simulink model "closedloop_3d"  (R2016b)
settings: Solver=FixedStepAuto  StartTime=0.0  StopTime=40  FixedStep=0.001  RelTol=1e-3
values from neighbouring files (symbols this model uses):
  C_psi = 3.1176e-5    (= 3.1176e-05)    [NL_1D_Model.m]    (also in NL_3D_Model.m)
  dead_time = 0.001    [NL_3D_Model.m]
  filter_select = 1    [NL_3D_Model.m]
  I_K_inv = inv(I_K)    [NL_3D_Model.m]
  I_R_inv = inv(I_R)    [NL_3D_Model.m]
  K = [ 0.0361, 1.0652, -1.1013, -0.6746, 0.3836, 0.1820, -0.0015, -0.0001, -0.0001 ... (first row only)    [NL_3D_Model.m]
  l_C = (l_M*m_r+l_AC*m_k)/m_g    [NL_1D_Model.m]    (also in NL_3D_Model.m = 0.066)
  m = m_r + m_k    (= 0.311)    [NL_1D_Model.m]    (also in NL_3D_Model.m = 1.532)
  T_comp = 2    [NL_3D_Model.m]
  Ta = 0.02    [NL_3D_Model.m]
  u_sat_on = true    [NL_3D_Model_u_limited.m]    (also in NL_3D_Model_u_limited_x_offset.m)
  x_0 = degtorad([3;0;0])    [NL_1D_Model.m]    (also in NL_3D_Model_u_limited.m = [x_0;zeros(6,1)]; NL_3D_Model_u_limited_x_offset.m = [x_0;zeros(6,1)])
  x_offset = zeros(9,1)    [NL_3D_Model_u_limited.m]    (also in NL_3D_Model_u_limited_x_offset.m = [0.05; 0.2; 0.5; zeros(6,1)])
libraries: vrlib x3, simulink x1
settings Model: Creator=michael  LastModifiedBy=michael

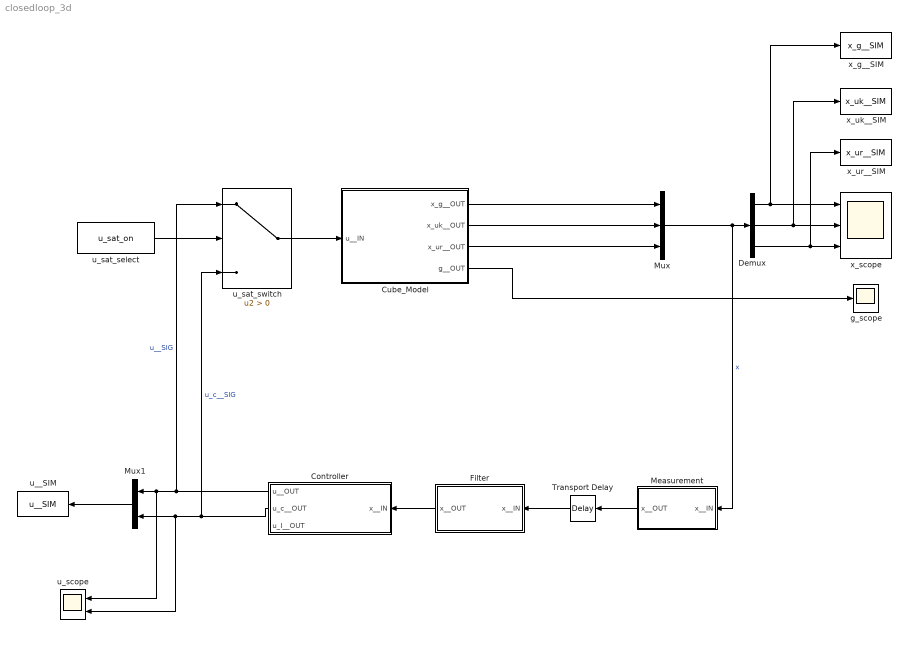
== system closedloop_3d ==
  Controller : Subsystem
  Cube_Model : Subsystem
  Demux : Demux  Outputs=3
  Filter : Subsystem
  Measurement : Subsystem
  Mux : Mux  Inputs=3
  Mux1 : Mux  Inputs=2
  Transport Delay : TransportDelay  DelayTime=dead_time  InitialOutput=x_0
  g_scope : Scope
  u__SIM : ToWorkspace  VariableName=u__SIM  SaveFormat=Timeseries  SampleTime=-1
  u_sat_select : Constant  Value=u_sat_on
  u_sat_switch : Switch  Criteria=u2 > Threshold
  u_scope : Scope  NumInputPorts=2
  x_g__SIM : ToWorkspace  VariableName=x_g__SIM  SaveFormat=Timeseries  SampleTime=-1
  x_scope : Scope  NumInputPorts=3
  x_uk__SIM : ToWorkspace  VariableName=x_uk__SIM  SaveFormat=Timeseries  SampleTime=-1
  x_ur__SIM : ToWorkspace  VariableName=x_ur__SIM  SaveFormat=Timeseries  SampleTime=-1
  wires:
  Cube_Model/1(x_g__OUT) -> Mux/1
  Cube_Model/2(x_uk__OUT) -> Mux/2
  Cube_Model/3(x_ur__OUT) -> Mux/3
  Mux/1 -> Measurement/1(x__IN), Demux/1  "x"
  Demux/3 -> x_ur__SIM/1, x_scope/3
  Demux/1 -> x_g__SIM/1, x_scope/1
  Demux/2 -> x_uk__SIM/1, x_scope/2
  Cube_Model/4(g__OUT) -> g_scope/1
  u_sat_select/1 -> u_sat_switch/2
  Mux1/1 -> u__SIM/1
  Controller/1(u__OUT) -> u_sat_switch/1, u_scope/1, Mux1/1  "u__SIG"
  Controller/2(u_c__OUT) -> u_sat_switch/3, u_scope/2, Mux1/2  "u_c__SIG"
  Filter/1(x__OUT) -> Controller/1(x__IN)
  Measurement/1(x__OUT) -> Transport Delay/1
  Transport Delay/1 -> Filter/1(x__IN)
  u_sat_switch/1 -> Cube_Model/1(u__IN)

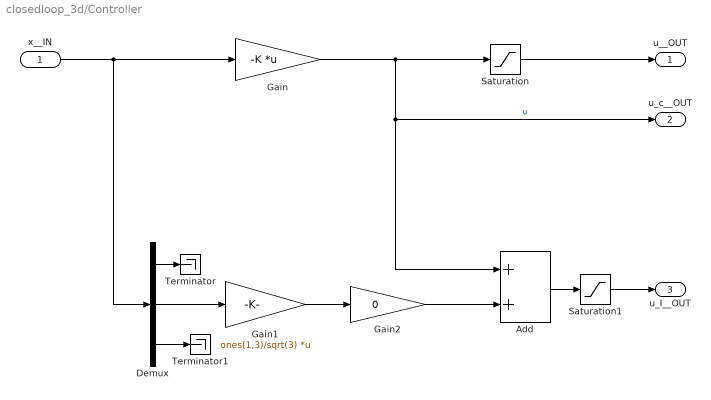
== system closedloop_3d/Controller ==
  x__IN : Inport  SampleTime=Ta
  Add : Sum
  Demux : Demux  Outputs=3
  Gain : Gain  Gain=-K  Multiplication=Matrix(K*u) (u vector)
  Gain1 : Gain  Gain=ones(1,3)/sqrt(3)  Multiplication=Matrix(K*u) (u vector)
  Gain2 : Gain  Gain=0
  Saturation : Saturate  UpperLimit=0.11  LowerLimit=-0.11
  Saturation1 : Saturate  UpperLimit=0.11  LowerLimit=-0.11
  Terminator : Terminator
  Terminator1 : Terminator
  u__OUT : Outport
  u_c__OUT : Outport  Port=2
  u_I__OUT : Outport  Port=3
  wires:
  x__IN/1 -> Demux/1, Gain/1
  Gain/1 -> Add/1, u_c__OUT/1, Saturation/1  "u"
  Saturation/1 -> u__OUT/1
  Demux/2 -> Gain1/1
  Demux/1 -> Terminator/1
  Gain1/1 -> Gain2/1
  Add/1 -> Saturation1/1
  Gain2/1 -> Add/2
  Saturation1/1 -> u_I__OUT/1
  Demux/3 -> Terminator1/1

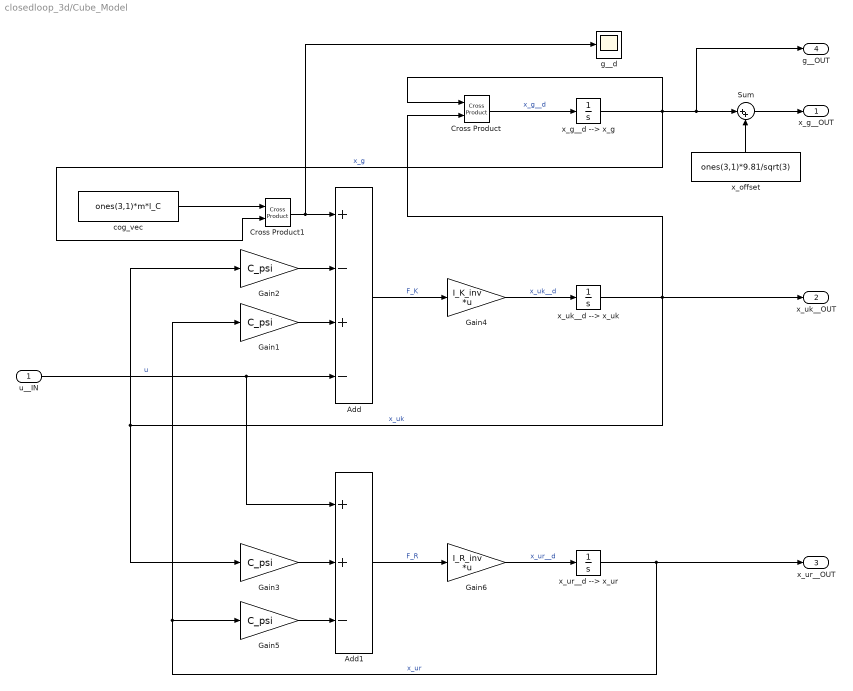
== system closedloop_3d/Cube_Model ==
  u__IN : Inport
  Add : Sum  Inputs=+-+-
  Add1 : Sum  Inputs=++-
  Cross Product : vrlib/Utilities/Cross Product
  Cross Product1 : vrlib/Utilities/Cross Product
  Gain{1..3,5} (4 alike) : Gain  Gain=C_psi
  Gain4 : Gain  Gain=I_K_inv  Multiplication=Matrix(K*u) (u vector)
  Gain6 : Gain  Gain=I_R_inv  Multiplication=Matrix(K*u) (u vector)
  Sum : Sum  Inputs=|++
  cog_vec : Constant  Value=ones(3,1)*m*l_C
  g__d : Scope
  x_g__d --> x_g : Integrator  InitialCondition=x_0(1:3)
  x_offset : Constant  Value=ones(3,1)*9.81/sqrt(3)
  x_uk__d --> x_uk : Integrator  InitialCondition=x_0(4:6)
  x_ur__d --> x_ur : Integrator  InitialCondition=x_0(7:9)
  x_g__OUT : Outport
  x_uk__OUT : Outport  Port=2
  x_ur__OUT : Outport  Port=3
  g__OUT : Outport  Port=4
  wires:
  Add/1 -> Gain4/1  "F_K"
  Gain5/1 -> Add1/3
  Gain4/1 -> x_uk__d --> x_uk/1  "x_uk__d"
  Gain1/1 -> Add/3
  Gain2/1 -> Add/2
  u__IN/1 -> Add1/1, Add/4  "u"
  Gain3/1 -> Add1/2
  x_ur__d --> x_ur/1 -> x_ur__OUT/1, Gain1/1, Gain5/1  "x_ur"
  Gain6/1 -> x_ur__d --> x_ur/1  "x_ur__d"
  Add1/1 -> Gain6/1  "F_R"
  x_g__d --> x_g/1 -> Cross Product1/2, g__OUT/1, Sum/1, Cross Product/1  "x_g"
  x_uk__d --> x_uk/1 -> x_uk__OUT/1, Cross Product/2, Gain3/1, Gain2/1  "x_uk"
  Cross Product/1 -> x_g__d --> x_g/1  "x_g__d"
  Sum/1 -> x_g__OUT/1
  x_offset/1 -> Sum/2
  cog_vec/1 -> Cross Product1/1
  Cross Product1/1 -> g__d/1, Add/1

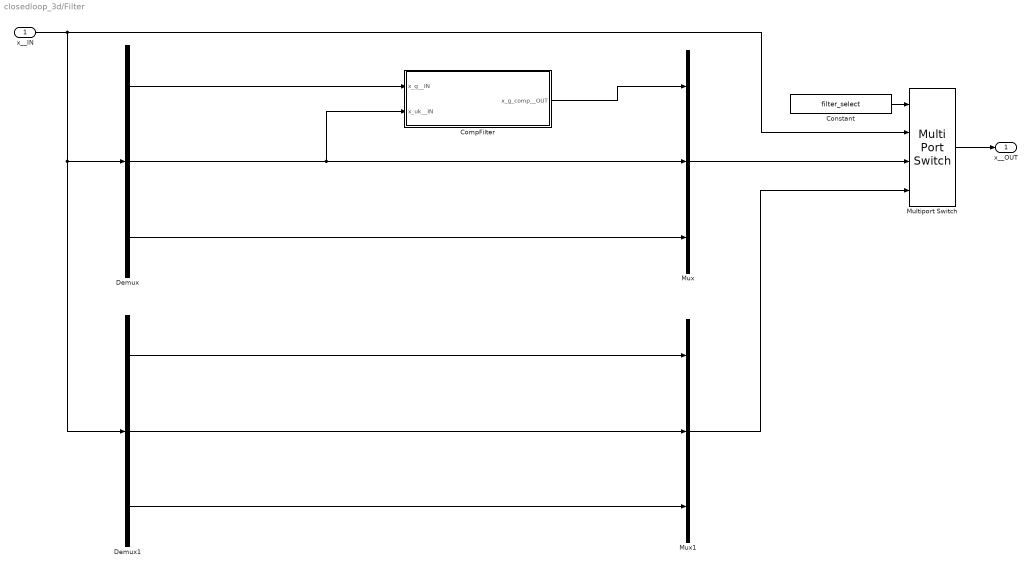
== system closedloop_3d/Filter ==
  x__IN : Inport  SampleTime=0.02
  CompFilter : Subsystem
  Constant : Constant  Value=filter_select
  Demux : Demux  Outputs=3
  Demux1 : Demux  Outputs=3
  Multiport Switch : MultiPortSwitch  DataPortOrder=Zero-based contiguous
  Mux : Mux  Inputs=3
  Mux1 : Mux  Inputs=3
  x__OUT : Outport
  wires:
  x__IN/1 -> Multiport Switch/2, Demux1/1, Demux/1
  Demux/2 -> Mux/2, CompFilter/2(x_uk__IN)
  Mux/1 -> Multiport Switch/3
  Demux/3 -> Mux/3
  CompFilter/1(x_g_comp__OUT) -> Mux/1
  Demux/1 -> CompFilter/1(x_g__IN)
  Demux1/1 -> Mux1/1
  Demux1/2 -> Mux1/2
  Demux1/3 -> Mux1/3
  Constant/1 -> Multiport Switch/1
  Multiport Switch/1 -> x__OUT/1
  Mux1/1 -> Multiport Switch/4

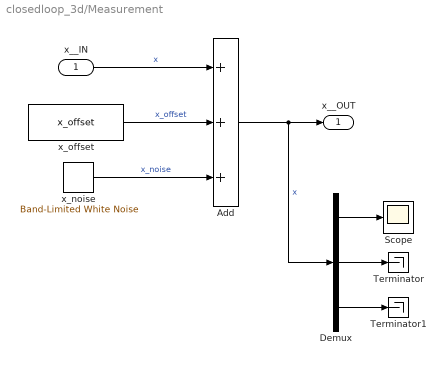
== system closedloop_3d/Measurement ==
  x__IN : Inport
  Add : Sum  Inputs=+++
  Demux : Demux  Outputs=3
  Scope : Scope
  Terminator : Terminator
  Terminator1 : Terminator
  x_noise : simulink/Sources/Band-Limited White Noise  Cov=x_noise  Ts=Ta  seed=[23341, 12324, 12341, 0, 0, 0, 0, 0, 0]
  x_offset : Constant  Value=x_offset
  x__OUT : Outport
  wires:
  x__IN/1 -> Add/1  "x"
  Add/1 -> Demux/1, x__OUT/1  "x"
  x_offset/1 -> Add/2  "x_offset"
  x_noise/1 -> Add/3  "x_noise"
  Demux/1 -> Scope/1
  Demux/2 -> Terminator/1
  Demux/3 -> Terminator1/1

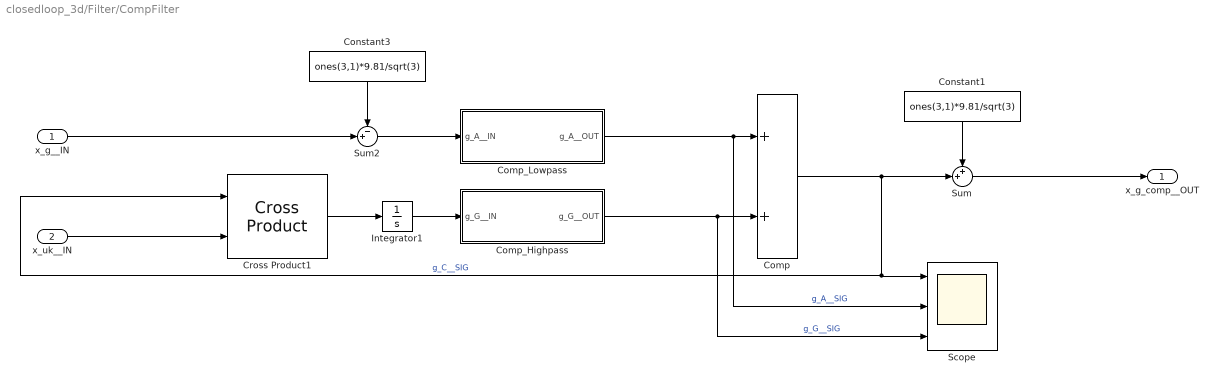
== system closedloop_3d/Filter/CompFilter ==
  x_g__IN : Inport
  x_uk__IN : Inport  Port=2
  Comp : Sum
  Comp_Highpass : Subsystem
  Comp_Lowpass : Subsystem
  Constant1 : Constant  Value=ones(3,1)*9.81/sqrt(3)
  Constant3 : Constant  Value=ones(3,1)*9.81/sqrt(3)
  Cross Product1 : vrlib/Utilities/Cross Product
  Integrator1 : Integrator  InitialCondition=x_0(1:3)
  Scope : Scope  NumInputPorts=3
  Sum : Sum  Inputs=++|
  Sum2 : Sum  Inputs=-+|
  x_g_comp__OUT : Outport
  wires:
  x_uk__IN/1 -> Cross Product1/2
  Comp_Lowpass/1(g_A__OUT) -> Scope/2, Comp/1  "g_A__SIG"
  Cross Product1/1 -> Integrator1/1
  Comp/1 -> Sum/2, Cross Product1/1, Scope/1  "g_C__SIG"
  Comp_Highpass/1(g_G__OUT) -> Scope/3, Comp/2  "g_G__SIG"
  Integrator1/1 -> Comp_Highpass/1(g_G__IN)
  x_g__IN/1 -> Sum2/2
  Sum2/1 -> Comp_Lowpass/1(g_A__IN)
  Constant3/1 -> Sum2/1
  Sum/1 -> x_g_comp__OUT/1
  Constant1/1 -> Sum/1

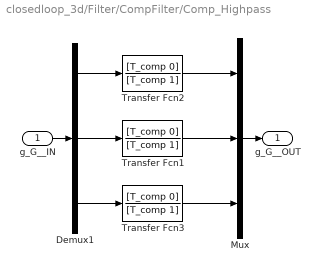
== system closedloop_3d/Filter/CompFilter/Comp_Highpass ==
  g_G__IN : Inport
  Demux1 : Demux  Outputs=3
  Mux : Mux  Inputs=3
  Transfer Fcn1 : TransferFcn  Numerator=[T_comp 0]  Denominator=[T_comp 1]
  Transfer Fcn2 : TransferFcn  Numerator=[T_comp 0]  Denominator=[T_comp 1]
  Transfer Fcn3 : TransferFcn  Numerator=[T_comp 0]  Denominator=[T_comp 1]
  g_G__OUT : Outport
  wires:
  Demux1/3 -> Transfer Fcn3/1
  g_G__IN/1 -> Demux1/1
  Transfer Fcn3/1 -> Mux/3
  Demux1/2 -> Transfer Fcn1/1
  Transfer Fcn1/1 -> Mux/2
  Mux/1 -> g_G__OUT/1
  Demux1/1 -> Transfer Fcn2/1
  Transfer Fcn2/1 -> Mux/1

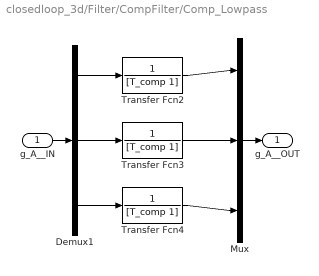
== system closedloop_3d/Filter/CompFilter/Comp_Lowpass ==
  g_A__IN : Inport
  Demux1 : Demux  Outputs=3
  Mux : Mux  Inputs=3
  Transfer Fcn2 : TransferFcn  Denominator=[T_comp 1]
  Transfer Fcn3 : TransferFcn  Denominator=[T_comp 1]
  Transfer Fcn4 : TransferFcn  Denominator=[T_comp 1]
  g_A__OUT : Outport
  wires:
  Transfer Fcn2/1 -> Mux/1
  Demux1/1 -> Transfer Fcn2/1
  Mux/1 -> g_A__OUT/1
  Transfer Fcn3/1 -> Mux/2
  Demux1/2 -> Transfer Fcn3/1
  Transfer Fcn4/1 -> Mux/3
  g_A__IN/1 -> Demux1/1
  Demux1/3 -> Transfer Fcn4/1
